simulink model "MR_Sensor_Angle_Calibration_Calculation"  (R2024a)
settings: Solver=FixedStepDiscrete  StartTime=0.0  StopTime=Inf  FixedStep=0.001  RelTol=1e-3
libraries: simulink x3
settings Model: Creator=Yuchen Lin  LastModifiedBy=Kylo_Ren
settings SolverCC: AlgebraicLoopSolver=TrustRegion
settings DataIOCC: ReturnWorkspaceOutputs=off
settings DebuggingCC: UnconnectedInputMsg=warning  UnconnectedOutputMsg=warning  UnconnectedLineMsg=warning  ArithmeticOperatorsInVariantConditions=warning
settings ModelReferenceCC: EnableRefExpFcnMdlSchedulingChecks=on
settings SFSimCC: SimUseLocalCustomCode=off  CustomCodeUndefinedFunction=UseInterfaceOnly
settings RTWCC: RTWUseLocalCustomCode=off  GPUComputeCapability=3.5
settings ConfigComp: CovBoundaryAbsTol=1.0e-5

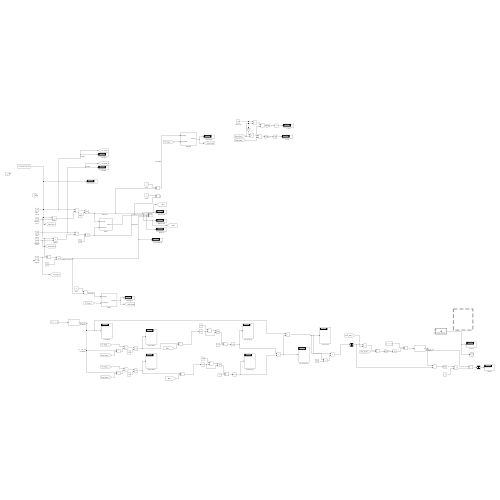
[thumbnail: Simulink's stored preview of the top-level diagram]
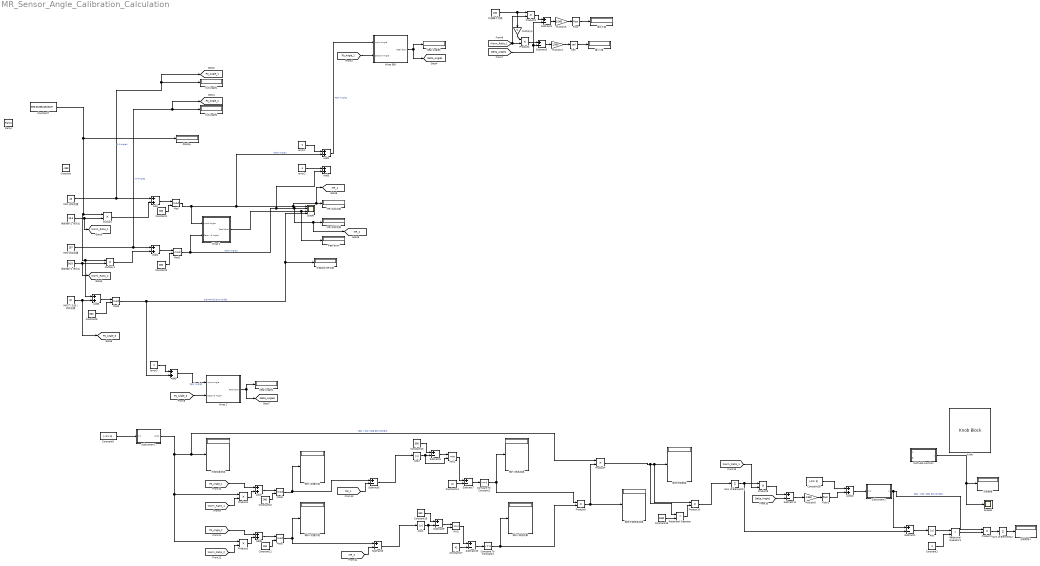
== system MR_Sensor_Angle_Calibration_Calculation ==
  0点Angle1 : Display
  0点Angle2 : Display
  Abs : Abs  SaturateOnIntegerOverflow=off
  Abs1 : Abs  SaturateOnIntegerOverflow=off
  Abs2 : Abs  SaturateOnIntegerOverflow=off
  Add{,1..3,6..10} (9 alike) : Sum
  Ceil : Rounding  Operator=ceil
  Compare To Constant1 : simulink/Logic and Bit Operations/Compare To Constant  relop=<=  const=0  OutDataTypeStr=boolean
  Compare To Constant2 : simulink/Logic and Bit Operations/Compare To Constant  relop=<=  const=0  OutDataTypeStr=boolean
  Constant : Constant  Value=-999
  Constant1 : Constant  Value=3
  Constant{2..3,8,10..11,13,16} (7 alike) : Constant  Value=360
  Constant14 : Constant  Value=41
  Constant17 : Constant  Value=41
  Constant18 : Constant  Value=[-3:1: 3]
  Constant19 : Constant  Value=1080
  Constant7 : Constant  Value=695.6106811523437
  Constant9 : Constant  Value=[-3:1: 3]
  Display : Display
  Floor : Rounding
  Floor1 : Rounding
  Ideal Angle1 : Display
  Ideal Angle3 : Display
  Knob : KnobBlock  ScaleMin=-1080  ScaleMax=1080
  MATLAB Function : MATLAB Function  TreatAsAtomicUnit=on
  MR1 初始位置 : Constant  Value=43
  MR1实际读数 : Display
  MR2 初始位置 : Constant  Value=287
  MR2实际读数 : Display
  MR3 （主轴） 初始位置 : Constant  Value=97
  Min1 : MinMax  Inputs=2
  Min2 : MinMax  Inputs=2
  Mod : Math  Operator=mod  SignedPower=on
  Mod1 : Math  Operator=mod  SignedPower=on
  Mod3 : Math  Operator=mod  SignedPower=on
  Mod4 : Math  Operator=mod
  Mod5 : Math  Operator=mod
  Multiply : Product
  Multiply1 : Product
  Multiply3 : Gain  Gain=1/360
  Multiply4 : Gain  Gain=-1
  Multiply5 : Gain  Gain=1/360
  Multiply6 : Gain  Gain=1/360
  Product{1..7,9..10} (9 alike) : Product
  Ramp : simulink/Sources/Ramp  slope=1  start=0  InitialOutput=-1080
  Real error : Display
  Relational Operator : RelationalOperator  Operator=<  OutDataTypeStr=boolean  RndMeth=Simplest  InputSameDT=off
  Relational Operator1 : RelationalOperator  Operator=<  OutDataTypeStr=boolean  RndMeth=Simplest  InputSameDT=off
  Scope : Scope  NumInputPorts=4
  Scope1 : Scope
  Subsystem1 : Subsystem
  Subsystem2 : Subsystem
  Subtract{1,3..11} (10 alike) : Sum  Inputs=+-
  Sum of Elements1 : Sum  Inputs=+
  Sum of Elements2 : Sum  Inputs=+
  Wrap 1 : Subsystem
  Wrap 2 : Subsystem
  Wrap 360 : Subsystem
  error1 : Constant  Value=-1
  error2 : Constant  Value=-1
  error3 : Constant  Value=2
  主轴位置待选 : Display
  主轴实际MR读数 : Display
  主轴角度 : Display
  主轴角度1 : Display
  最大K值 : Display
  最小K值 : Display
  最终主轴筛选结果 : Display
  最终主轴角度 : Display
  机械最大范围 : Constant  Value=180
  蜗杆1位置待选 : Display
  蜗杆1筛选结果 : Display
  蜗杆2位置待选 : Display
  蜗杆2筛选结果 : Display
  "蜗轮蜗杆1 传动比 " : Constant  Value=19.5
  "蜗轮蜗杆2 传动比 " : Constant  Value=56/3
  tag scope: Delta_Angle1=global, Delta_Angle3=global, MR_1=global, MR_2=global, P0_Angle_1=global, P0_Angle_2=global, P0_Angle_3=global, Worm_Ratio_1=global, Worm_Ratio_2=global
  wires:
  "蜗轮蜗杆1 传动比 "/1 -> [Worm_Ratio_1], Multiply/2
  Multiply/1 -> Add/2
  "蜗轮蜗杆2 传动比 "/1 -> [Worm_Ratio_2], Multiply1/2
  Multiply1/1 -> Add1/2
  Add/1 -> Mod/1
  Constant2/1 -> Mod/2
  Mod/1 -> Wrap 1/1(Input Angle), Add2/2, [MR_1], MR1实际读数/1, Scope/1  "Ideal Angle1"
  Add1/1 -> Mod1/1
  Constant3/1 -> Mod1/2
  Mod1/1 -> Wrap 1/2(Second Angle), Add3/2, [MR_2], MR2实际读数/1, Scope/2  "Ideal Angle2"
  Constant7/1 -> Multiply/1, Add6/1, Multiply1/1, Display/1
  error1/1 -> Add2/1
  error2/1 -> Add3/1
  MR2 初始位置/1 -> Add1/1, [P0_Angle_2], 0点Angle2/1  "0点Angle2"
  MR1 初始位置/1 -> [P0_Angle_1], 0点Angle1/1, Add/1  "0点Angle1"
  Add2/1 -> Wrap 360/1(Input Angle)  "Real Angle1"
  Wrap 1/1(Real Error) -> Real error/1, Scope/3
  [P0_Angle_1] -> Wrap 360/2(Second Angle)
  Wrap 360/1(Real Error) -> [Delta_Angle1], Ideal Angle3/1
  机械最大范围/1 -> Multiply4/1, Product3/1
  [Worm_Ratio_1] -> Product2/2, Product3/2
  Product2/1 -> Subtract3/1
  [Delta_Angle1] -> Subtract4/2, Subtract3/2
  Subtract3/1 -> Multiply3/1
  Multiply3/1 -> Ceil/1
  Multiply4/1 -> Product2/1
  Product3/1 -> Subtract4/1
  Subtract4/1 -> Multiply5/1
  Multiply5/1 -> Floor/1
  Floor/1 -> 最大K值/1
  Ceil/1 -> 最小K值/1
  MR3 （主轴） 初始位置/1 -> [P0_Angle_3], Add6/2
  Add6/1 -> Mod3/1
  Constant8/1 -> Mod3/2
  Mod3/1 -> 主轴实际MR读数/1, Scope/4, Add9/2  "主轴MR3没加error的读数"
  [P0_Angle_3] -> Wrap 2/2(Second Angle)
  Wrap 2/1(Real Error) -> [Delta_Angle3], Ideal Angle1/1
  Constant9/1 -> Subsystem1/1(In1)
  Constant10/1 -> Mod4/2
  Product4/1 -> Add7/2
  [Worm_Ratio_1] -> Product4/2
  Add7/1 -> Mod4/1
  [P0_Angle_1] -> Add7/1
  Mod4/1 -> 蜗杆1位置待选/1, Subtract5/1
  Subsystem1/1(Out1) -> Product5/1, Product4/1, Product7/1, 主轴位置待选/1  "蜗轮（主轴）角度 通过MR3算出"
  [P0_Angle_2] -> Add8/1
  Constant11/1 -> Mod5/2
  Add8/1 -> Mod5/1
  Product5/1 -> Add8/2
  [Worm_Ratio_2] -> Product5/2
  [MR_1] -> Subtract5/2
  Constant13/1 -> Subtract6/1
  Abs2/1 -> Min1/2, Subtract6/2
  Subtract6/1 -> Min1/1
  Subtract7/1 -> Compare To Constant1/1
  Min1/1 -> Subtract7/1
  Constant14/1 -> Subtract7/2
  Compare To Constant1/1 -> Product6/1, 蜗杆1筛选结果/1
  [MR_2] -> Subtract8/2
  Min2/1 -> Subtract10/1
  Subtract10/1 -> Compare To Constant2/1
  Abs1/1 -> Min2/2, Subtract9/2
  Constant16/1 -> Subtract9/1
  Mod5/1 -> Subtract8/1, 蜗杆2位置待选/1
  Subtract9/1 -> Min2/1
  Compare To Constant2/1 -> 蜗杆2筛选结果/1, Product6/2
  Constant17/1 -> Subtract10/2
  Product6/1 -> Product7/2, 最终主轴筛选结果/1
  Product7/1 -> Product10/1, 最终主轴角度/1, Relational Operator/1
  MATLAB Function/1(y) -> Scope1/1, 主轴角度/1
  error3/1 -> Add9/1
  Add9/1 -> Wrap 2/1(Input Angle)  "Real Angle2"
  Constant18/1 -> Add10/1
  Sum of Elements1/1 -> Subtract1/2, Product9/1
  [Worm_Ratio_1] -> Product9/2
  [Delta_Angle1] -> Subtract11/2
  Product9/1 -> Subtract11/1
  Floor1/1 -> Add10/2
  Multiply6/1 -> Floor1/1
  Subtract11/1 -> Multiply6/1
  Add10/1 -> Subsystem2/1(In1)
  Subsystem2/1(A) -> Subtract1/1, Product1/1  "蜗轮（主轴）角度 通过MR1算出"
  Constant19/1 -> Relational Operator/2
  Relational Operator/1 -> Product10/2
  Product10/1 -> Sum of Elements1/1
  Subtract5/1 -> Abs2/1
  Subtract8/1 -> Abs1/1
  Subtract1/1 -> Abs/1
  Abs/1 -> Relational Operator1/1
  Constant1/1 -> Relational Operator1/2
  Relational Operator1/1 -> Product1/2
  Product1/1 -> Sum of Elements2/1
  Sum of Elements2/1 -> 主轴角度1/1

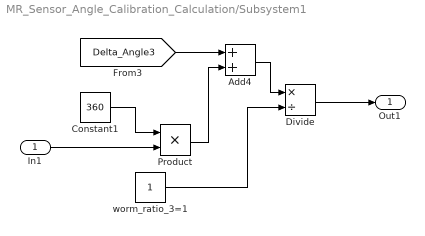
== system MR_Sensor_Angle_Calibration_Calculation/Subsystem1 ==
  In1 : Inport
  Add4 : Sum
  Constant1 : Constant  Value=360
  Divide : Product  Inputs=*/
  Product : Product
  worm_ratio_3=1 : Constant
  Out1 : Outport
  wires:
  [Delta_Angle3] -> Add4/1
  Constant1/1 -> Product/1
  In1/1 -> Product/2
  Add4/1 -> Divide/1
  Divide/1 -> Out1/1
  worm_ratio_3=1/1 -> Divide/2
  Product/1 -> Add4/2

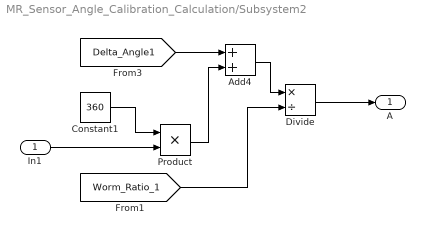
== system MR_Sensor_Angle_Calibration_Calculation/Subsystem2 ==
  In1 : Inport
  Add4 : Sum
  Constant1 : Constant  Value=360
  Divide : Product  Inputs=*/
  Product : Product
  A : Outport
  wires:
  [Delta_Angle1] -> Add4/1
  Constant1/1 -> Product/1
  In1/1 -> Product/2
  Add4/1 -> Divide/1
  Divide/1 -> A/1
  [Worm_Ratio_1] -> Divide/2
  Product/1 -> Add4/2

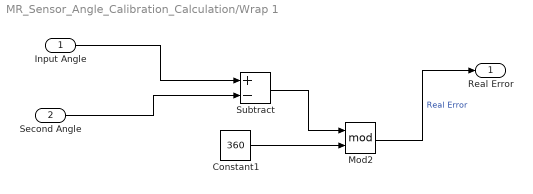
== system MR_Sensor_Angle_Calibration_Calculation/Wrap 1 ==
  Input Angle : Inport
  Second Angle : Inport  Port=2
  Constant1 : Constant  Value=360
  Mod2 : Math  Operator=mod
  Subtract : Sum  Inputs=+-
  Real Error : Outport
  wires:
  Subtract/1 -> Mod2/1
  Constant1/1 -> Mod2/2
  Mod2/1 -> Real Error/1  "Real Error"
  Input Angle/1 -> Subtract/1
  Second Angle/1 -> Subtract/2

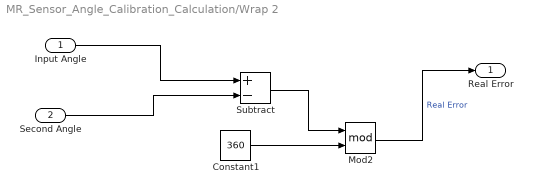
== system MR_Sensor_Angle_Calibration_Calculation/Wrap 2 ==
  Input Angle : Inport
  Second Angle : Inport  Port=2
  Constant1 : Constant  Value=360
  Mod2 : Math  Operator=mod
  Subtract : Sum  Inputs=+-
  Real Error : Outport
  wires:
  Subtract/1 -> Mod2/1
  Constant1/1 -> Mod2/2
  Mod2/1 -> Real Error/1  "Real Error"
  Input Angle/1 -> Subtract/1
  Second Angle/1 -> Subtract/2

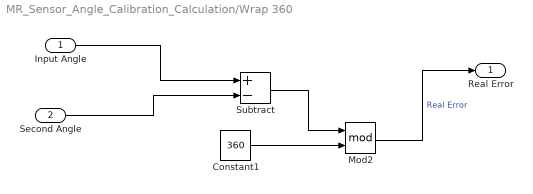
== system MR_Sensor_Angle_Calibration_Calculation/Wrap 360 ==
  Input Angle : Inport
  Second Angle : Inport  Port=2
  Constant1 : Constant  Value=360
  Mod2 : Math  Operator=mod
  Subtract : Sum  Inputs=+-
  Real Error : Outport
  wires:
  Subtract/1 -> Mod2/1
  Constant1/1 -> Mod2/2
  Mod2/1 -> Real Error/1  "Real Error"
  Input Angle/1 -> Subtract/1
  Second Angle/1 -> Subtract/2

== matlab function MR_Sensor_Angle_Calibration_Calculation/MATLAB Function ==
  data: A input; y output size=[1 3]; B input
function y = match_nonzero(A, B)
    tol = 3;

    temp = zeros(max(length(A),length(B)));

    k = 1;

    for i = 1:length(temp)
        if abs(A(i)) > 1e-2
            for j = 1:length(B)
                if abs(B(j)) > 1e-2 && abs(A(i)-B(j)) < tol
                    temp(k) = A(i);
                    k = k + 1;
                    break;
                end
            end
        end
    end

y = temp(1:k-1);
